simulink subsystem "GCRF_to_ICRF"  (R2023b)
settings: Solver=VariableStepAuto  StartTime=0.0  StopTime=10.0  RelTol=1e-3
libraries: aerolibutil x1
settings Model: DefaultTestHarness=ITRF_to_GCRF_Harness1  Creator=laura  LastModifiedBy=laura
settings OptimizationCC: ReuseModelBlockBuffer=off

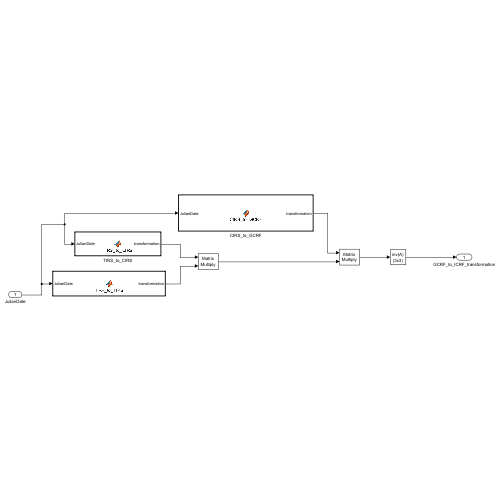
[thumbnail: Simulink's stored preview of the top-level diagram]
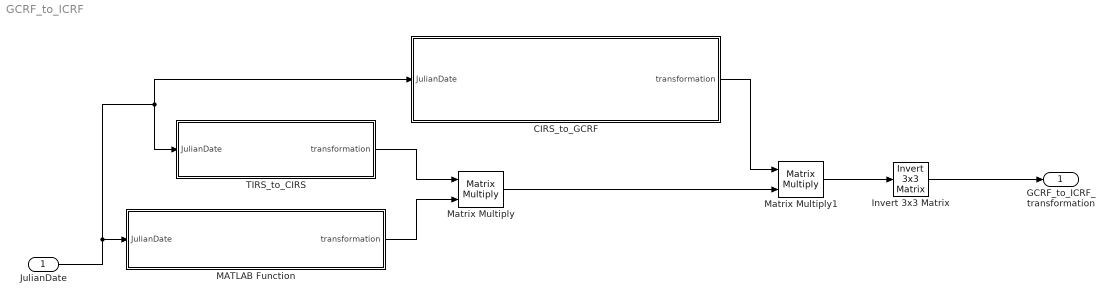
== system GCRF_to_ICRF ==
  JulianDate : Inport
  CIRS_to_GCRF : MATLAB Function  TreatAsAtomicUnit=on
  Invert 3x3 Matrix : aerolibutil/Invert  3x3 Matrix
  MATLAB Function : MATLAB Function  TreatAsAtomicUnit=on
  Matrix Multiply : Product  Multiplication=Matrix(*)
  Matrix Multiply1 : Product  Multiplication=Matrix(*)
  TIRS_to_CIRS : MATLAB Function  TreatAsAtomicUnit=on
  GCRF_to_ICRF_transformation : Outport
  wires:
  MATLAB Function/1(transformation) -> Matrix Multiply/2
  TIRS_to_CIRS/1(transformation) -> Matrix Multiply/1
  JulianDate/1 -> CIRS_to_GCRF/1(JulianDate), TIRS_to_CIRS/1(JulianDate), MATLAB Function/1(JulianDate)
  CIRS_to_GCRF/1(transformation) -> Matrix Multiply1/1
  Matrix Multiply/1 -> Matrix Multiply1/2
  Matrix Multiply1/1 -> Invert 3x3 Matrix/1
  Invert 3x3 Matrix/1 -> GCRF_to_ICRF_transformation/1

== matlab function GCRF_to_ICRF/MATLAB Function ==
  data: transformation output; JulianDate input
function transformation = ITRF_to_TIRS(JulianDate)

Julian_centuries = (JulianDate - 2451545) / 36525;
s_prime = -0.000047 * 0.0002778 * Julian_centuries; % s' is the TIO locator

MJD = JulianDate - 2400000.5;
A = 2 * pi * (MJD - 60257) / 365.25;
C = 2 * pi * (MJD - 60257) / 435;

% x_p and y_p are the predicted values for the International Reference Pole
% (IRP), based on the prediction model from 2023/11/11
x_p = 0.1444 + 0.0434*cos(A) - 0.0794*sin(A);
x_p = x_p + 0.0781*cos(C) - 0.0325*sin(C);
y_p = 0.3537 - 0.0690*cos(A) - 0.0446*sin(A);
y_p = y_p - 0.0325*cos(C) - 0.0781*sin(C);

% Arcseconds to degrees
x_p = x_p * 0.0002778;     
y_p = y_p * 0.0002778;     

R_x = rotx(y_p);
R_y = roty(x_p); 
R_z = rotz(-s_prime);

transformation = R_z * R_y * R_x;

== matlab function GCRF_to_ICRF/TIRS_to_CIRS ==
  data: transformation output; JulianDate input
function transformation = TIRS_to_CIRS(JulianDate)

Earth_rotation_angle = 2*pi* (0.779057273264 + 1.00273781191135448*(JulianDate - 2451545));

transformation = rotz(-Earth_rotation_angle);

== matlab function GCRF_to_ICRF/CIRS_to_GCRF ==
  data: transformation output; JulianDate input
function transformation = CIRS_to_GCRF(JulianDate)

    XValuesTable = my_readtable("reference_frames\tablea.dat");

    rowNumber = 1;

    JulianCenturies = (JulianDate - 2451545) / 36525;

    X = - 0.016617 + 2004.191898*JulianCenturies - 0.4297829*JulianCenturies^2 ...
        - 0.19861834 * JulianCenturies^3 + 0.000007578*JulianCenturies^4 + 0.0000059285*JulianCenturies^5;
    
    for i = 1:1306
        a_pi = calculateTrigArgument(XValuesTable{rowNumber, :}, JulianCenturies);
        X = X + XValuesTable{rowNumber, 4} * sin(a_pi) + XValuesTable{rowNumber, 5} * cos(a_pi);
        rowNumber = rowNumber + 1;
    end    
    
    for i = 1:253
        a_pi = calculateTrigArgument(XValuesTable{rowNumber, :}, JulianCenturies);
        X = X + (XValuesTable{rowNumber, 4} * sin(a_pi) + XValuesTable{rowNumber, 5} * cos(a_pi)) * JulianCenturies;
        rowNumber = rowNumber + 1;
    end

    for i = 1:36
        a_pi = calculateTrigArgument(XValuesTable{rowNumber, :}, JulianCenturies);
        X = X + (XValuesTable{rowNumber, 4} * sin(a_pi) + XValuesTable{rowNumber, 5} * cos(a_pi)) * JulianCenturies^2;
        rowNumber = rowNumber + 1;
    end

    for i = 1:4
        a_pi = calculateTrigArgument(XValuesTable{rowNumber, :}, JulianCenturies);
        X = X + (XValuesTable{rowNumber, 4} * sin(a_pi) + XValuesTable{rowNumber, 5} * cos(a_pi)) * JulianCenturies^3;
        rowNumber = rowNumber + 1;
    end

    a_pi = calculateTrigArgument(XValuesTable{rowNumber, :}, JulianCenturies);
    X = X + (XValuesTable{rowNumber, 4} * sin(a_pi) + XValuesTable{rowNumber, 5} * cos(a_pi)) * JulianCenturies^4;

    % Calculate Y

    YValuesTable = my_readtable("reference_frames\tableb.dat");
    rowNumber = 1;

    Y = -0.006951 - 0.025896*JulianCenturies - 22.407274*JulianCenturies^2 ...
        + 0.00190059*JulianCenturies^3 + 0.001112526*JulianCenturies^4 + 0.0000001358*JulianCenturies^5;
    
    for i = 1:962
        a_pi = calculateTrigArgument(YValuesTable{rowNumber, :}, JulianCenturies);
        Y = Y + YValuesTable{rowNumber, 4} * sin(a_pi) + YValuesTable{rowNumber, 5} * cos(a_pi);
        rowNumber = rowNumber + 1;
    end    
    
    for i = 1:277
        a_pi = calculateTrigArgument(YValuesTable{rowNumber, :}, JulianCenturies);
        Y = Y + (YValuesTable{rowNumber, 4} * sin(a_pi) + YValuesTable{rowNumber, 5} * cos(a_pi)) * JulianCenturies;
        rowNumber = rowNumber + 1;
    end

    for i = 1:30
        a_pi = calculateTrigArgument(YValuesTable{rowNumber, :}, JulianCenturies);
       Y = Y + (YValuesTable{rowNumber, 4} * sin(a_pi) + YValuesTable{rowNumber, 5} * cos(a_pi)) * JulianCenturies^2;
        rowNumber = rowNumber + 1;
    end

    for i = 1:5
        a_pi = calculateTrigArgument(YValuesTable{rowNumber, :}, JulianCenturies);
        Y = Y + (YValuesTable{rowNumber, 4} * sin(a_pi) + YValuesTable{rowNumber, 5} * cos(a_pi)) * JulianCenturies^3;
        rowNumber = rowNumber + 1;
    end

    a_pi = calculateTrigArgument(YValuesTable{rowNumber, :}, JulianCenturies);
    Y = Y + (YValuesTable{rowNumber, 4} * sin(a_pi) + YValuesTable{rowNumber, 5} * cos(a_pi)) * JulianCenturies^4;
    
    % Calculate s
    sValuesTable = my_readtable("reference_frames\tablec.dat");
    rowNumber = 1;

    s = -(X*Y)/2;
    s = s + 0.000094 + 0.00380865*JulianCenturies - 0.00012268*JulianCenturies^2 ...
        - 0.07257411*JulianCenturies^3 + 0.00002798*JulianCenturies^4 + 0.00001562*JulianCenturies^5;
    
    for i = 1:33
        a_pi = calculateTrigArgument(sValuesTable{rowNumber, :}, JulianCenturies);
        s = s + sValuesTable{rowNumber, 4} * sin(a_pi) + sValuesTable{rowNumber, 5} * cos(a_pi);
        rowNumber = rowNumber + 1;
    end    
    
    for i = 1:3
        a_pi = calculateTrigArgument(sValuesTable{rowNumber, :}, JulianCenturies);
        s = s + (sValuesTable{i, 4} * sin(a_pi) + sValuesTable{i, 5} * cos(a_pi)) * JulianCenturies;
        rowNumber = rowNumber + 1;
    end

    for i = 1:25
        a_pi = calculateTrigArgument(sValuesTable{rowNumber, :}, JulianCenturies);
        s = s + (sValuesTable{i, 4} * sin(a_pi) + sValuesTable{i, 5} * cos(a_pi)) * JulianCenturies^2;
        rowNumber = rowNumber + 1;
    end

    for i = 1:4
        a_pi = calculateTrigArgument(sValuesTable{rowNumber, :}, JulianCenturies);
        s = s + (sValuesTable{i, 4} * sin(a_pi) + sValuesTable{i, 5} * cos(a_pi)) * JulianCenturies^3;
        rowNumber = rowNumber + 1;
    end

        a_pi = calculateTrigArgument(sValuesTable{rowNumber, :}, JulianCenturies);
        s = s + (sValuesTable{i, 4} * sin(a_pi) + sValuesTable{i, 5} * cos(a_pi)) * JulianCenturies^4;

    a = 1/2 + 1/8 * (X^2+Y^2);
    
    PN = [ (1-a*X^2) (-a*X*Y) (X); (-a*X*Y) (1-a*Y^2) (Y); (-X) (-Y) (1-a*(X^2 +Y^2))];
    R_z = rotz(s);

    transformation = PN*R_z;
end


function trigArgument = calculateTrigArgument(tableRow, JulianCenturies)
    trigArgument = 0;
    trigArgument = trigArgument + tableRow(6) * (485868.249036 + ...
        1717915923.2178 * JulianCenturies + 31.8792*JulianCenturies^2 + 0.051635*JulianCenturies^3 - ...
        0.00024470 * JulianCenturies^4);

    trigArgument = trigArgument + tableRow(7) * (1287104.79305 + ...
        129596581.0481*JulianCenturies - 0.5532*JulianCenturies^2 + 0.000136*JulianCenturies^3 ...
        - 0.00001149*JulianCenturies^4);
    
    trigArgument = trigArgument + tableRow(8) * (335779.526232 + ...
        1739527262.8478*JulianCenturies - 12.7512*JulianCenturies^2 - 0.001037*JulianCenturies^3 + ...
        0.00000417*JulianCenturies^4);
   
    trigArgument = trigArgument + tableRow(9) * (1072260.70369 + ...
        1602961601.2090*JulianCenturies - 6.3706*JulianCenturies^2 + 0.006593*JulianCenturies^3 - ...
        0.00003169*JulianCenturies^4);

    trigArgument = trigArgument + tableRow(10) * (450160.398036 - ...
        6962890.5431*JulianCenturies + 7.4722*JulianCenturies^2 + 0.007702*JulianCenturies^3 - ...
        0.00005939*JulianCenturies^4);
    
    trigArgument = trigArgument + tableRow(11) * (4.402608842 + 2608.7903141574*JulianCenturies);
    trigArgument = trigArgument + tableRow(12) * (3.176146697 + 1021.3285546211*JulianCenturies);
    trigArgument = trigArgument + tableRow(13) * (1.753470314 + 628.3075849991*JulianCenturies);
    trigArgument = trigArgument + tableRow(14) * (6.203480913 + 334.0612426700*JulianCenturies);
    trigArgument = trigArgument + tableRow(15) * (0.599546497 + 52.9690962641*JulianCenturies);
    trigArgument = trigArgument + tableRow(16) * (0.874016757 + 21.3299104960*JulianCenturies);
    trigArgument = trigArgument + tableRow(17) * (5.481293872 + 7.4781598567*JulianCenturies);
    trigArgument = trigArgument + tableRow(18) * (5.311886287 + 3.8133035638*JulianCenturies);
    trigArgument = trigArgument + tableRow(19) * (0.02438175*JulianCenturies + 0.00000538691*JulianCenturies^2);

end

function T = my_readtable(filename)

    f = fopen(filename,"r");
    size = [19 Inf];
    data = fscanf(f,'%f', size);
    data = transpose(data);
    
    % Construct the table
    T = array2table(data, 'VariableNames', {'N','j','i','asji','acji','nl','nlprime','nF','nD','nOm','nLMe','nLV','nLE','nLMa','nLJ','nLS','nLU','nLN','npa'});
    fclose(f);

end
